simulink model "pd_plus_testings_7DOF_alternative"  (R2022b)
settings: Solver=ode4  StartTime=0.0  StopTime=101  FixedStep=1e-3  RelTol=1e-3
InitFcn:
  | parameters_7dof;
undefined symbols (not defined in the file): param_robot, q_0
(part 4 of 7)

== matlab function pd_plus_testings_7DOF_alternative/7 DOF Model/Mass Matrix1 ==
  data: q_state input; M output
function M = Franka_MassmMatrix(q_state)
% Author: TU Wien, ACIN Robotics group
% Optimized and generated from Maple

  M = zeros(7,7);
  t437 = q_state(6);
  t423 = sin(t437);
  t430 = cos(t437);
  t552 = 0.60149e-1 * t423 - 0.14117e-1 * t430;
  t302 = t552 + 0.384e0;
  t439 = q_state(4);
  t425 = sin(t439);
  t270 = t302 * t425;
  t440 = q_state(3);
  t433 = cos(t440);
  t327 = 0.60149e-1 * t430 + 0.14117e-1 * t423;
  t438 = q_state(5);
  t424 = sin(t438);
  t431 = cos(t438);
  t218 = t327 * t424 + 0.10517e-1 * t431;
  t426 = sin(t440);
  t484 = t218 * t426;
  t432 = cos(t439);
  t732 = 0.10517e-1 * t424;
  t495 = -t327 * t431 + t732;
  t965 = 0.825e-1 + t495;
  t974 = t432 * t965;
  t1004 = t484 + (t270 + t974) * t433;
  t436 = q_state(7);
  t422 = sin(t436);
  t355 = 0.12009367848960000000000000000000e-2 * t422;
  t275 = t355 + 0.63347540234880000000000000000000e-1;
  t429 = cos(t436);
  t379 = 0.29704261916160000000000000000000e-2 * t429;
  t190 = -t379 - t275;
  t361 = 0.55042935974400000000000000000000e-3 * t422;
  t408 = t422 ^ 2;
  t791 = 0.13297872941088000000000000000000e-4 * t408 + t361;
  t184 = 0.57804776249276620000000000000000e-2 + t791;
  t415 = t429 ^ 2;
  t375 = 0.24076459055801420000000000000000e-2 * t415;
  t516 = -t375 + t184;
  t615 = 0.79021743663150400000000000000000e-3 * t422;
  t865 = (-0.13614453378240000000000000000000e-2 + t615) * t429;
  t119 = t865 - t516;
  t992 = t119 * t423;
  t944 = t992 + t190;
  t1003 = t430 * t944;
  t232 = 0.10517000000000000000000000000000e-1 * t422 - 0.42520000000000000000000000000000e-2 * t429;
  t733 = 0.61597e-1 * t423;
  t556 = -0.10517e-1 * t429 - 0.4252e-2 * t422;
  t312 = -t556 + 0.88e-1;
  t854 = t312 * t430;
  t477 = t733 + t854;
  t955 = t424 * t477;
  t924 = -t232 * t431 + t955;
  t871 = t232 * t424;
  t818 = t430 * t431;
  t969 = -t312 * t818 - t431 * t733 + 0.825e-1;
  t126 = -t871 + t969;
  t476 = t312 * t423 - 0.61597e-1 * t430;
  t968 = 0.384e0 + t476;
  t948 = t425 * t968;
  t532 = -0.825e-1 + t948;
  t98 = t126 * t432 + t532;
  t1001 = t426 * t924 + t433 * t98;
  t975 = t965 * t425;
  t441 = q_state(2);
  t434 = cos(t441);
  t806 = t434 * t432;
  t427 = sin(t441);
  t822 = t427 * t433;
  t306 = t425 * t822 + t806;
  t857 = t306 * t430;
  t831 = t426 * t427;
  t807 = t434 * t425;
  t810 = t432 * t433;
  t298 = -0.1e1 * t427 * t810 + t807;
  t956 = t298 * t431;
  t201 = t424 * t831 + t956;
  t884 = t201 * t423;
  t979 = -0.1e1 * t884 + t857;
  t410 = t424 ^ 2;
  t417 = t431 ^ 2;
  t841 = t424 * t431;
  t672 = 0.4234e-2 * t841;
  t999 = 0.29474e-1 * t410 + 0.35549e-1 * t417 + t672 + 0.25853e-1;
  t998 = 0.28179e-1;
  t492 = 0.98827089590400000000000000000000e-3 * t422 + 0.52129746651620000000000000000000e-1;
  t198 = 0.24444132201840000000000000000000e-2 * t429 + t492;
  t997 = t198 * t423;
  t416 = t430 ^ 2;
  t523 = 0.33449653235675560000000000000000e-2 * t429 - 0.10967182128164640000000000000000e-2 * t422;
  t189 = 0.11022068765350630000000000000000e-1 + t523;
  t845 = t423 * t430;
  t779 = t189 * t845;
  t996 = (t119 * t416 - t779 + 0.23330419227411030000000000000000e-2) * t410;
  t364 = 0.25801376238000000000000000000000e-3 * t422;
  t290 = 0.13609823097337500000000000000000e-1 + t364;
  t384 = 0.63817750210500000000000000000000e-3 * t429;
  t939 = t384 + t290;
  t165 = t939 * t425;
  t995 = -t165 + t198;
  t590 = 0.10967182128164640000000000000000e-2 * t429;
  t324 = t423 * t590;
  t524 = -0.15804348732630080000000000000000e-2 * t415 - 0.13614453378240000000000000000000e-2 * t422 + 0.5826996021941340000000000000000e-3;
  t143 = (0.48418875570424600000000000000000e-2 * t422 + 0.55042935974400000000000000000000e-3) * t429 + t524;
  t959 = t143 * t430;
  t627 = -0.3030488946654060e-2 - t959;
  t994 = t324 + t627;
  t351 = 0.29704261916160000000000000000000e-2 * t422;
  t566 = 0.23898270415101870000000000000000e-1 - t351;
  t573 = 0.12009367848960000000000000000000e-2 * t429;
  t193 = t566 + t573;
  t376 = 0.79021743663150400000000000000000e-3 * t415;
  t292 = -0.68072266891200000000000000000000e-3 * t422 + 0.29134980109706700000000000000000e-3;
  t274 = 0.24209437785212300000000000000000e-2 * t422 + 0.27521467987200000000000000000000e-3;
  t866 = t274 * t429;
  t984 = t292 + t866;
  t967 = -t376 + t984;
  t987 = t967 * t423;
  t479 = -t987 - t193;
  t993 = t432 - 0.1e1;
  t610 = 0.33449653235675560000000000000000e-2 * t422;
  t105 = -(0.187138194629210e-3 + t610) * t423 - t994;
  t910 = t105 * t417;
  t991 = t218 * t433;
  t832 = t425 * t433;
  t741 = 0.4252e-2 * t429;
  t557 = 0.10517e-1 * t422 - t741;
  t513 = t557 * t431;
  t457 = t513 - t955;
  t990 = t457 * t426;
  t588 = 0.14820000000000000000000000000000e-2 * t429;
  t323 = t423 * t588;
  t612 = 0.23920000000000000000000000000000e-2 * t422;
  t849 = t422 * t429;
  t544 = 0.49780000000000000000000000000000e-2 * t849;
  t618 = 0.17120000000000000000000000000000e-2 * t415;
  t177 = t544 - 0.14600000000000000000000000000000e-2 - t618;
  t897 = t177 * t430;
  t799 = t897 - (0.682e-3 + t612) * t423;
  t930 = -t323 + 0.4234e-2 + t799;
  t989 = t841 * t930;
  t848 = t423 * t424;
  t988 = t848 * t967;
  t986 = t967 * t424;
  t985 = t967 * t430;
  t972 = t375 + t865;
  t115 = (-0.89033153705875550000000000000000e-2 - t791 + t972) * t416;
  t803 = t115 - t779;
  t402 = 0.345563e0 * t425;
  t389 = -0.825e-1 + t402;
  t551 = 0.41065e-1 * t424 + 0.11953e-1 * t431;
  t303 = t551 + 0.825e-1;
  t858 = t303 * t432;
  t203 = t389 + t858;
  t233 = -0.41065000000000000000000000000000e-1 * t431 + 0.11953000000000000000000000000000e-1 * t424;
  t129 = t203 * t426 + t233 * t433;
  t983 = -0.32797153116247448000000000000000e-1 - t791 + t865;
  t442 = q_state(1);
  t435 = cos(t442);
  t805 = t434 * t435;
  t763 = t426 * t805;
  t428 = sin(t442);
  t820 = t428 * t433;
  t982 = -t763 - t820;
  t592 = 0.54835910640823200000000000000000e-3 * t429;
  t325 = t423 * t592;
  t644 = t325 + 0.2390110552949070e-2;
  t613 = 0.16724826617837780000000000000000e-2 * t422;
  t856 = (0.93569097314605e-4 + t613) * t423;
  t981 = t910 + t644 + t856;
  t371 = 0.56786982094425000000000000000000e-2 * t425;
  t980 = -0.1e1 * t371 + 0.26431758938496000000000000000000e-1 * t432 + 0.21751134959804000000000000000000e-1;
  t769 = t431 * t831;
  t861 = t298 * t424;
  t183 = t861 - 0.1e1 * t769;
  t978 = -t996 - 0.1e1 * t361;
  t860 = t302 * t432;
  t976 = t425 * t495 - t860;
  t360 = 0.63817750210500000000000000000000e-3 * t422;
  t594 = 0.25801376238000000000000000000000e-3 * t429;
  t491 = 0.55993270925625000000000000000000e-2 + t594;
  t194 = -t360 + t491;
  t169 = t194 * t432;
  t483 = t592 + t613;
  t208 = t483 + 0.93569097314605e-4;
  t877 = t208 * t430;
  t281 = 0.56786982094425000000000000000000e-2 * t423 - 0.12089329343850000000000000000000e-2;
  t242 = t281 * t432;
  t164 = t423 * t939;
  t748 = 0.825e-1 * t434;
  t824 = t427 * t425;
  t973 = t748 * t810 + 0.825e-1 * t824;
  t546 = 0.85600000000000000000000000000000e-3 * t849;
  t617 = 0.24890000000000000000000000000000e-2 * t415;
  t221 = t546 + t617;
  t462 = t221 - 0.27050000000000000000000000000000e-2;
  t175 = t221 + 0.28220000000000000000000000000000e-2;
  t899 = t175 * t416;
  t460 = t899 + t462;
  t380 = 0.23920000000000000000000000000000e-2 * t429;
  t614 = 0.14820000000000000000000000000000e-2 * t422;
  t522 = -t380 + t614;
  t223 = -0.218e-3 + t522;
  t778 = t223 * t845;
  t101 = t778 + t460;
  t545 = 0.24890000000000000000000000000000e-2 * t849;
  t619 = 0.85600000000000000000000000000000e-3 * t415;
  t174 = t545 - 0.73000000000000000000000000000000e-3 - t619;
  t591 = 0.74100000000000000000000000000000e-3 * t429;
  t543 = t423 * t591;
  t744 = -0.11960000000000000000000000000000e-2 * t422 - 0.341e-3;
  t736 = t744 * t423 + 0.3449e-2;
  t971 = t101 * t841 + t174 * t430 - t543 + t736;
  t321 = 0.17120000000000000000000000000000e-2 * t849;
  t373 = 0.49780000000000000000000000000000e-2 * t415;
  t794 = t321 + t373;
  t800 = -t899 - t778;
  t509 = -0.33106000000000000000000000000000e-1 + t794 + t800;
  t804 = (-t462 + t800) * t417 - t989;
  t970 = t509 + t804;
  t124 = t375 + t983;
  t508 = -0.8292e-2 + t614;
  t179 = 0.5644000000000000000000000000000e-2 + t794;
  t784 = t179 * t845;
  t377 = 0.47840000000000000000000000000000e-2 * t429;
  t611 = 0.29640000000000000000000000000000e-2 * t422;
  t224 = t611 - t377 - 0.436e-3;
  t873 = t224 * t416;
  t966 = -0.1e1 * t508 + t380 + t873 - 0.1e1 * t784;
  t964 = -0.1e1 * t380 + t508 + t784 - 0.1e1 * t873;
  t458 = -t424 * t557 - t431 * t477;
  t569 = 0.11357396418885000000000000000000e-1 * t423 - 0.24178658687700000000000000000000e-2;
  t480 = t371 - 0.21751134959804000000000000000000e-1 * t432;
  t963 = t480 - 0.26431758938496000000000000000000e-1;
  t962 = -0.50330438027992300000000000000000e0 - t997;
  t961 = 0.29682175996164750000000000000000e0 + t164;
  t958 = t194 * t431;
  t607 = 0.88000000000000000000000000000000e-1 * t423;
  t279 = 0.38400000000000000000000000000000e0 + t607;
  t957 = t279 * t426;
  t548 = -0.104419e0 * t432 + 0.5317e-1 * t425;
  t953 = t427 * t548;
  t699 = 0.345563e0 * t432;
  t859 = t303 * t425;
  t626 = -t699 + t859;
  t952 = t427 * t626;
  t322 = t429 * t615;
  t816 = t430 * t433;
  t765 = t433 * t805;
  t830 = t426 * t428;
  t562 = t432 * (t765 - 0.1e1 * t830);
  t199 = 0.12763550042100000000000000000000e-2 * t429 + 0.51602752476000000000000000000000e-3 * t422 + 0.27219646194675000000000000000000e-1;
  t950 = (t199 * t430 + t569) * t431;
  t949 = (t626 - 0.316e0) * t434;
  t879 = t968 * t432;
  t277 = -t360 + 0.55993270925625000000000000000000e-2;
  t946 = (t277 + t594) * t432;
  t550 = -0.41065e-1 * t431 + 0.11953e-1 * t424;
  t945 = t550 * t426;
  t409 = t423 ^ 2;
  t365 = 0.31228377456598930000000000000000e-2 * t409;
  t789 = t365 - t322;
  t135 = 0.25022978729410880000000000000000e-2 * t415 + 0.81354094419858000000000000000000e-4 * t408 - t789 - 0.6284682367054690000000000000000e-3;
  t943 = t115 + t135;
  t229 = -0.825e-1 + t270;
  t941 = t229 + t974;
  t942 = t433 * t941 + t484;
  t382 = 0.13614453378240000000000000000000e-2 * t429;
  t790 = -t361 - t382;
  t388 = 0.54835910640823200000000000000000e-3 * t433;
  t595 = 0.24444132201840000000000000000000e-2 * t426;
  t938 = t388 + t595;
  t937 = -0.59408523832320000000000000000000e-2 * t422 + 0.24018735697920000000000000000000e-2 * t429 + 0.47796540830203740000000000000000e-1 + t143 * t423;
  t936 = -0.1e1 * t375 - 0.26431758938496000000000000000000e-1 * t430 - t983;
  t935 = t422 * t732 - t424 * t741 - t969;
  t353 = 0.15804348732630080000000000000000e-2 * t422;
  t287 = 0.24018735697920000000000000000000e-2 * t422 + 0.12669508046976000000000000000000e0;
  t464 = t287 + 0.59408523832320000000000000000000e-2 * t429;
  t885 = t199 * t423;
  t934 = ((0.66899306471351120000000000000000e-2 * t429 - 0.21934364256329280000000000000000e-2 * t422 + 0.22044137530701260000000000000000e-1) * t416 + ((0.48152918111602840000000000000000e-2 * t415 + (t353 - 0.27228906756480000000000000000000e-2) * t429 - 0.26595745882176000000000000000000e-4 * t408 - 0.11008587194880000000000000000000e-2 * t422 - 0.11560955249855324000000000000000e-1) * t423 - t464) * t430 - 0.52863517876992000000000000000000e-1 * t423 - 0.8968493211292842000000000000000e-2 - t523) * t431 + 0.27752814537092170000000000000000e0 + t885;
  t702 = 0.249498e0 * t427;
  t730 = 0.39252e-1 * t426;
  t933 = -t434 * t730 + t702;
  t673 = 0.7735484874e-2 * t429;
  t677 = 0.3127439544e-2 * t422;
  t932 = t673 + t677;
  t931 = 0.88e-1 * t430 + t733;
  t891 = t939 * t432;
  t927 = -t891 + t199;
  t354 = 0.12763550042100000000000000000000e-2 * t422;
  t291 = 0.11198654185125000000000000000000e-1 - t354;
  t593 = 0.51602752476000000000000000000000e-3 * t429;
  t926 = -0.1e1 * t593 - 0.1e1 * t291;
  t703 = 0.104419e0 * t425;
  t549 = 0.5317e-1 * t432 + t703;
  t304 = t549 - 0.825e-1;
  t502 = t304 * t426;
  t720 = 0.27454e-1 * t433;
  t925 = (t502 + t720) * t435;
  t923 = 0.735522e0 * t428;
  t701 = 0.735522e0 * t430;
  t381 = 0.16724826617837780000000000000000e-2 * t429;
  t362 = 0.54835910640823200000000000000000e-3 * t422;
  t567 = 0.44842466056464210000000000000000e-2 - t362;
  t191 = t381 + t567;
  t600 = 0.12089329343850000000000000000000e-2 * t425;
  t374 = 0.24209437785212300000000000000000e-2 * t415;
  t793 = t322 + t374;
  t898 = (0.31228377456598930000000000000000e-2 + t793) * t409;
  t922 = (t191 * t432 + t980 * t423 + t600 - 0.46305794820080000000000000000000e-2) * t431 + (0.23126197987767817000000000000000e-1 + t898) * t425;
  t706 = 0.27518e-1 * t428;
  t711 = 0.39252e-1 * t435;
  t921 = t435 * t702 + (-t434 * t711 - t706) * t426;
  t844 = t423 * t431;
  t920 = t174 * t844 + 0.8641e-2;
  t919 = -t177 * t844 - 0.17282e-1;
  t918 = 0.1225946e1 * t129;
  t352 = 0.24444132201840000000000000000000e-2 * t422;
  t489 = 0.98827089590400000000000000000000e-3 * t429 + 0.21447119530300000000000000000000e-1;
  t185 = -t352 + t489;
  t280 = -0.21751134959804000000000000000000e-1 * t423 + 0.46305794820080000000000000000000e-2;
  t916 = t185 * t424 + (-0.1e1 * t198 * t430 + t280) * t431;
  t915 = 0.25801376238000000000000000000000e-3 * t425 - 0.98827089590400000000000000000000e-3;
  t909 = t930 * t417;
  t914 = -t425 * t909 - 0.12805000000000000000000000000000e-1;
  t103 = (-0.1e1 * t865 + t516) * t423 - t190;
  t911 = t103 * t430;
  t571 = t306 * t423;
  t883 = t201 * t430;
  t136 = t571 + t883;
  t906 = t136 * t422;
  t905 = t136 * t429;
  t900 = (-0.99560000000000000000000000000000e-2 * t849 + 0.34240000000000000000000000000000e-2 * t415 + 0.29200000000000000000000000000000e-2) * t430;
  t160 = t179 * t416;
  t896 = t183 * t422;
  t895 = t183 * t429;
  t893 = t185 * t432;
  t892 = (-0.60427308755286430000000000000000e-2 + t790) * t409;
  t167 = t189 * t416;
  t192 = 0.89166132435286430000000000000000e-2 - t790;
  t890 = t192 * t432;
  t889 = t193 * t432;
  t888 = t194 * t425;
  t370 = 0.82500000000000000000000000000000e-1 * t425;
  t285 = 0.38400000000000000000000000000000e0 - t370;
  t197 = -t285 - 0.31600000000000000000000000000000e0 * t432;
  t887 = t197 * t430;
  t886 = t198 * t432;
  t202 = t483 + 0.9356909731460500000000000000000e-4;
  t882 = t202 * t424;
  t881 = t202 * t430;
  t880 = t203 * t433;
  t482 = -t590 - t610;
  t207 = -t482 + 0.187138194629210e-3;
  t878 = t207 * t423;
  t481 = -t588 - t612;
  t875 = (-t481 + 0.682e-3) * t430;
  t874 = t223 * t416;
  t225 = -t591 + t744;
  t872 = t225 * t430;
  t869 = t233 * t426;
  t272 = 0.18713819462921000000000000000000e-3 + t610;
  t868 = t272 * t423;
  t867 = t274 * t423;
  t864 = t277 * t425;
  t863 = t287 * t423;
  t246 = t292 * t423;
  t293 = 0.9356909731460500000000000000000e-4 + t613;
  t862 = t293 * t433;
  t853 = (0.47840000000000000000000000000000e-2 * t422 + 0.1364e-2) * t423;
  t847 = t423 * t426;
  t846 = t423 * t429;
  t843 = t424 * t426;
  t842 = t424 * t430;
  t840 = t424 * t432;
  t839 = t424 * t433;
  t838 = t424 * t434;
  t837 = t425 * t423;
  t836 = t425 * t424;
  t835 = t425 * t426;
  t834 = t425 * t430;
  t833 = t425 * t431;
  t828 = t426 * t432;
  t827 = t426 * t433;
  t826 = t426 * t434;
  t825 = t426 * t435;
  t823 = t427 * t432;
  t819 = t428 * t434;
  t817 = t430 * t432;
  t815 = t430 * t434;
  t814 = t431 * t432;
  t813 = t431 * t434;
  t812 = t432 * t423;
  t811 = t432 * t425;
  t809 = t433 * t434;
  t808 = t433 * t435;
  t715 = 0.10517e-1 * t435;
  t665 = t426 * t715;
  t721 = 0.10517e-1 * t433;
  t257 = -t428 * t721 - t434 * t665;
  t650 = t433 * t715;
  t728 = 0.10517e-1 * t428;
  t260 = -t426 * t728 + t434 * t650;
  t662 = t427 * t715;
  t802 = (-t260 * t425 + t432 * t662) * t423 + t257 * t842;
  t738 = 0.4252e-2 * t435;
  t267 = t738 * t809 - 0.4252e-2 * t830;
  t670 = t427 * t738;
  t740 = 0.4252e-2 * t430;
  t801 = (-t267 * t425 + t432 * t670) * t423 + t982 * t424 * t740;
  t181 = t224 * t845;
  t798 = t160 + t181;
  t757 = 0.88e-1 * t435;
  t685 = t433 * t757;
  t759 = 0.88e-1 * t426;
  t687 = t428 * t759;
  t268 = -t434 * t685 + t687;
  t686 = t427 * t757;
  t797 = t268 * t425 + t432 * t686;
  t368 = 0.35079000000000000000000000000000e-3 * t424;
  t283 = -t368 - 0.92549600000000000000000000000000e-3;
  t796 = t283 * t432 + t368;
  t574 = 0.10517000000000000000000000000000e-1 * t435;
  t795 = t574 * t826 + 0.10517000000000000000000000000000e-1 * t820;
  t746 = 0.825e-1 * t435;
  t401 = t433 * t746;
  t347 = t434 * t401;
  t406 = 0.316e0 * t427;
  t400 = t435 * t406;
  t792 = t347 + t400;
  t749 = 0.825e-1 * t433;
  t396 = t427 * t749;
  t788 = -t396 + 0.316e0 * t434;
  t787 = -0.1e1 * t432 + 0.1e1;
  t786 = -0.1e1 * t321 - 0.1e1 * t373;
  t785 = t432 * t898;
  t783 = t433 * t167;
  t154 = t189 * t812;
  t782 = t225 * t842;
  t333 = -0.8074e-2 * t431 - 0.458e-3 * t424;
  t781 = t333 * t811;
  t780 = t175 * t845;
  t153 = (0.21800000000000000000000000000000e-3 - t522) * t845;
  t776 = t424 * t813;
  t773 = t189 * t837;
  t772 = t430 * t807;
  t771 = t425 * t806;
  t770 = t426 * t819;
  t768 = t430 * t814;
  t767 = t431 * t810;
  t766 = t428 * t809;
  t764 = t435 * t824;
  t753 = 0.825e-1 * t428;
  t683 = t426 * t753;
  t762 = t432 * t683 + t792;
  t761 = -t406 + t973;
  t760 = -t425 * t748 + t788;
  t756 = 0.428e-3 * t422;
  t755 = 0.109e-3 * t423;
  t754 = 0.384e0 * t425;
  t752 = 0.384e0 * t428;
  t751 = 0.428e-3 * t429;
  t750 = 0.109e-3 * t430;
  t747 = 0.384e0 * t434;
  t745 = 0.384e0 * t435;
  t742 = 0.4252e-2 * t427;
  t739 = 0.3495e-2 * t435;
  t317 = -0.74100000000000000000000000000000e-3 * t422 + 0.4146e-2;
  t366 = 0.26431758938496000000000000000000e-1 * t423;
  t148 = -t366 - t191;
  t735 = t148 + t167;
  t336 = t425 * t662;
  t734 = t260 * t432 + t336;
  t731 = 0.27454e-1 * t426;
  t729 = 0.61597e-1 * t426;
  t727 = 0.14117e-1 * t428;
  t726 = 0.27454e-1 * t428;
  t725 = 0.39252e-1 * t428;
  t724 = 0.60149e-1 * t428;
  t719 = 0.27518e-1 * t433;
  t718 = 0.39252e-1 * t433;
  t717 = 0.61597e-1 * t433;
  t716 = 0.10517e-1 * t434;
  t714 = 0.14117e-1 * t435;
  t713 = 0.27454e-1 * t435;
  t712 = 0.27518e-1 * t435;
  t710 = 0.60149e-1 * t435;
  t709 = 0.61597e-1 * t435;
  t125 = t924 * t433;
  t624 = -0.1e1 * t854 - t733;
  t707 = 0.735522e0 * (t126 * t828 + t426 * t532 - t125) * t435 + (t1001 * t434 - 0.1e1 * t406 + (-t879 + (0.825e-1 - 0.1e1 * t871 + t624 * t431) * t425) * t427) * t923;
  t328 = 0.2872e-1 * t434 + 0.3141e-2 * t427;
  t704 = 0.646926e0 * t328;
  t128 = -t880 + t869;
  t697 = 0.1225946e1 * (t128 * t434 + t406 + (-0.1e1 * t859 + t699) * t427) * t435 + t428 * t918;
  t144 = -t945 + t880;
  t696 = 0.1225946e1 * (t144 * t434 - t406 + t952) * t428 + t435 * t918;
  t645 = t860 - t975;
  t695 = 0.1666555e1 * (t645 + 0.316e0) * t434 + 0.1666555e1 * t942 * t427;
  t137 = t426 * t712 + t428 * t933 + t433 * t711 + t706 * t809;
  t692 = 0.3228604e1 * t137;
  t630 = t304 * t433 - t731;
  t691 = -0.3587895e1 * t630 * t427 + 0.3587895e1 * (t548 - 0.316e0) * t434;
  t397 = t428 * t406;
  t680 = t426 * t746;
  t689 = t428 * t973 + t432 * t680 - t397;
  t681 = t433 * t747;
  t344 = t425 * t681;
  t688 = t344 + t761;
  t684 = t426 * t752;
  t682 = t428 * t748;
  t399 = t427 * t745;
  t679 = 0.3127439544e-2 * t279;
  t678 = 0.7735484874e-2 * t279;
  t676 = 0.3127439544e-2 * t424;
  t675 = 0.7735484874e-2 * t424;
  t674 = 0.3127439544e-2 * t429;
  t671 = t426 * t742;
  t669 = 0.15592e-1 * t811;
  t668 = 0.10517e-1 * t831;
  t667 = t428 * t729;
  t664 = t427 * t727;
  t663 = t427 * t724;
  t661 = t427 * t714;
  t660 = t427 * t710;
  t659 = t427 * t709;
  t658 = t428 * t716;
  t657 = t434 * t727;
  t656 = t434 * t724;
  t655 = t434 * t714;
  t654 = t434 * t712;
  t653 = t434 * t710;
  t652 = t434 * t709;
  t649 = 0.735522e0 * t832;
  t648 = t399 * t432 + t425 * t684 + t762;
  t642 = (0.76800000000000000000000000000000e0 * t423 + 0.17600000000000000000000000000000e0) * t673;
  t641 = t432 * t679;
  t286 = 0.31600000000000000000000000000000e0 - t370;
  t640 = t286 * t673;
  t639 = t344 * t428 + t745 * t835 + t689;
  t638 = t347 - t683;
  t637 = t765 - t830;
  t636 = t770 - t808;
  t635 = t735 + t1003;
  t632 = t770 - 0.1e1 * t808;
  t629 = -0.1e1 * t820 - 0.1e1 * t763;
  t628 = -0.1e1 * t766 - 0.1e1 * t825;
  t625 = t426 * t682 - t401;
  t623 = 0.7902174366315040000000000000000e-3 * t415;
  t622 = 0.2420943778521230000000000000000e-2 * t415;
  t621 = 0.5483591064082320000000000000000e-3 * t433;
  t616 = 0.28220000000000000000000000000000e-2 * t416;
  t609 = 0.14600000000000000000000000000000e-2 * t423;
  t608 = 0.49096519673609460000000000000000e-2 * t423;
  t606 = 0.86765250000000000000000000000000e-3 * t424;
  t605 = 0.42520000000000000000000000000000e-2 * t424;
  t604 = 0.49096519673609460000000000000000e-2 * t424;
  t602 = 0.54835910640823200000000000000000e-3 * t425;
  t601 = 0.63817750210500000000000000000000e-3 * t425;
  t598 = 0.25801376238000000000000000000000e-3 * t426;
  t597 = 0.63817750210500000000000000000000e-3 * t426;
  t596 = 0.16724826617837780000000000000000e-2 * t426;
  t589 = 0.11960000000000000000000000000000e-2 * t429;
  t586 = 0.54835910640823200000000000000000e-3 * t430;
  t585 = 0.16724826617837780000000000000000e-2 * t430;
  t584 = 0.11357396418885000000000000000000e-1 * t430;
  t583 = 0.54835910640823200000000000000000e-3 * t431;
  t582 = 0.25801376238000000000000000000000e-3 * t432;
  t581 = 0.54835910640823200000000000000000e-3 * t432;
  t580 = 0.63817750210500000000000000000000e-3 * t432;
  t579 = 0.16724826617837780000000000000000e-2 * t432;
  t578 = 0.49096519673609460000000000000000e-2 * t432;
  t577 = 0.10517000000000000000000000000000e-1 * t432;
  t572 = 0.21751134959804000000000000000000e-1 * t430;
  t570 = t322 - 0.60029938106866070000000000000000e-2;
  t568 = 0.12089329343850000000000000000000e-2 * t993;
  t563 = t432 * t632;
  t561 = -0.1e1 * t364 - 0.13609823097337500000000000000000e-1;
  t560 = t431 * t944 + t882;
  t559 = 0.2872e-1 * t427 - 0.3141e-2 * t434;
  t555 = t424 * t628;
  t554 = t425 * t629;
  t553 = t629 * t432;
  t547 = -t719 + t730;
  t542 = t423 * t598;
  t541 = t423 * t597;
  t540 = 0.49096519673609460000000000000000e-2 * t834;
  t539 = t423 * t581;
  t538 = t423 * t579;
  t537 = t431 * t578;
  t531 = t432 * t625 + t636 * t754 - t625;
  t162 = (-t427 * t746 - t435 * t681 + t684) * t425;
  t530 = (t399 - t638) * t432 + t162 + t400 + t638;
  t529 = 0.56786982094425000000000000000000e-2 * t787;
  t282 = -0.37417600000000000000000000000000e-3 + t606;
  t528 = t282 * t432 - t606;
  t519 = -0.1e1 * t384 + t561;
  t518 = t423 * t544;
  t507 = t366 + t381 + 0.44842466056464210000000000000000e-2 - t167 - 0.1e1 * t362;
  t506 = t376 - 0.1e1 * t866;
  t505 = -0.29640000000000000000000000000000e-2 * t846 + 0.8468e-2;
  t504 = -t589 + t780;
  t501 = (-t891 + t939) * t431 + t154;
  t500 = -0.65933151443131591200000000000000e0 - t642;
  t106 = t987 + (t293 + t592) * t430;
  t497 = t504 - t874;
  t494 = -t433 * t549 + t731;
  t490 = 0.11198654185125000000000000000000e-1 + t593;
  t487 = t425 * t551 - t699;
  t216 = t427 * t547 + 0.249498e0 * t434;
  t486 = t376 * t423 - 0.23898270415101870000000000000000e-1;
  t485 = t354 - t490;
  t236 = 0.16724826617837780000000000000000e-2 * t433 + 0.98827089590400000000000000000000e-3 * t426;
  t474 = t432 * t551 + t389;
  t473 = (0.12009367848960000000000000000000e-2 + t867) * t429 + t246 - t486;
  t470 = -(0.2489553776598930000000000000000e-3 + t793) * t416 + 0.23330419227411030000000000000000e-2 * t410 + 0.48418875570424600000000000000000e-2 * t415;
  t468 = 0.42520000000000000000000000000000e-2 * t982;
  t466 = -t432 * t678 + t601 - 0.24444132201840000000000000000000e-2;
  t463 = (0.104419e0 * t427 - 0.5317e-1 * t809) * t432 + (-0.104419e0 * t809 - 0.5317e-1 * t427) * t425;
  t461 = 0.46305794820080000000000000000000e-2 * t432 - t567 - t600;
  t459 = -t221 + 0.31784000000000000000000000000000e-1 + t798 + t804;
  t456 = t434 * t630 + t953;
  t455 = t425 * t552 + t432 * t495 - 0.825e-1;
  t454 = t945 + (-t402 - t858) * t433;
  t453 = t426 * t474 + t433 * t550;
  t452 = -t458 - 0.825e-1;
  t451 = t426 * t455 - t991;
  t450 = t487 * t427 + (t433 * t474 - t945) * t434;
  t449 = t425 * t458 - t879;
  t448 = t425 * t476 + t432 * t458 - 0.825e-1;
  t447 = (0.229e-3 + t872) * t431 + (-0.1e1 * t874 - 0.1e1 * t317 + t504) * t424 - t920;
  t446 = t976 * t427 + (t433 * t455 + t484) * t434;
  t445 = t426 * t448 + t433 * t457;
  t444 = t990 + (t432 * t452 - t948) * t433;
  t443 = t449 * t427 + (t433 * t448 - t990) * t434;
  t419 = t433 ^ 2;
  t418 = t432 ^ 2;
  t412 = t426 ^ 2;
  t411 = t425 ^ 2;
  t393 = t428 * t720;
  t385 = 0.21751134959804000000000000000000e-1 * t431;
  t372 = 0.54835910640823200000000000000000e-3 * t426;
  t348 = t425 * t686;
  t338 = t425 * t670;
  t337 = t433 * t654;
  t335 = t425 * t659;
  t332 = -0.8074e-2 * t424 + 0.458e-3 * t431;
  t319 = 0.458e-3 + t609;
  t310 = t434 * t713 - t753;
  t309 = t434 * t746 + t726;
  t308 = t434 * t726 + t746;
  t307 = t682 - t713;
  t300 = t574 * t824;
  t299 = t618 * t848;
  t288 = 0.82500000000000000000000000000000e-1 * t993;
  t284 = -0.31600000000000000000000000000000e0 * t425 + 0.82500000000000000000000000000000e-1;
  t269 = -t434 * t687 + t685;
  t265 = -t742 * t810 + 0.4252e-2 * t807;
  t264 = t433 * t709 - t434 * t667;
  t263 = -t433 * t658 - t665;
  t262 = -t426 * t652 - t428 * t717;
  t261 = t433 * t652 - t667;
  t259 = -t426 * t727 + t433 * t655;
  t258 = -t426 * t724 + t433 * t653;
  t256 = t426 * t655 + t433 * t727;
  t255 = t426 * t653 + t433 * t724;
  t254 = t426 * t714 + t433 * t657;
  t253 = -t426 * t710 - t433 * t656;
  t252 = t426 * t658 - t650;
  t251 = -t426 * t657 + t433 * t714;
  t250 = -t426 * t656 + t433 * t710;
  t249 = t425 * t716 - t721 * t823;
  t248 = t293 * t426;
  t245 = t290 * t425;
  t241 = t281 * t425;
  t234 = -t381 + t362;
  t231 = -0.12150e-1 * t841 - 0.4234e-2 * t410 + 0.4234e-2 * t417;
  t220 = t435 * t559 - 0.3495e-2 * t428;
  t213 = t285 * t673;
  t196 = -0.26431758938496000000000000000000e-1 * t425 - 0.56786982094425000000000000000000e-2 * t993;
  t188 = t286 + 0.38400000000000000000000000000000e0 * t432;
  t171 = t202 * t431;
  t170 = t464 * t423;
  t149 = -t197 + t607;
  t130 = t967 * t812;
  t127 = (-0.68072266891200000000000000000000e-3 * t429 - 0.27521467987200000000000000000000e-3 * t422 - 0.49096519673609460000000000000000e-2) * t430 + t234 * t423;
  t117 = (t261 * t425 + 0.88e-1 * t424 * t629 - t432 * t659) * t430;
  t108 = 0.42340000000000000000000000000000e-2 + t897 - t323 + (-0.68200000000000000000000000000000e-3 - t612) * t423;
  t107 = -t351 + t473;
  t91 = ((-0.68072266891200000000000000000000e-3 * t423 + t585 - 0.29704261916160000000000000000000e-2) * t429 + (-0.27521467987200000000000000000000e-3 * t423 - t586 - 0.12009367848960000000000000000000e-2) * t422 - t608) * t424 + (-0.25801376238000000000000000000000e-3 * t423 + (-0.12009367848960000000000000000000e-2 * t430 - 0.54835910640823200000000000000000e-3) * t431) * t429 + (0.63817750210500000000000000000000e-3 * t423 + (0.29704261916160000000000000000000e-2 * t430 - 0.16724826617837780000000000000000e-2) * t431) * t422;
  t90 = -t135 - t803;
  t86 = 0.15592e-1 + t964 * t431 - 0.1e1 * t299 + (t875 + t518 - 0.1e1 * t319) * t424;
  t82 = t936 * t431 + (t519 - t986) * t430 + (-t190 * t431 + t882 - 0.56786982094425000000000000000000e-2) * t423;
  t79 = (t507 - t1003) * t424 + (t881 - t479) * t431;
  t78 = ((t234 * t430 + t279 * t932 + t608) * t431 + (0.28244044800000000000000000000000e0 * t232 * t430 - 0.1e1 * t483) * t424) * t425 - 0.1e1 * t578 * t430 - 0.1e1 * t429 * t538 + t422 * t539 - 0.735522e0 * t556 * t288 * t431 + (t422 * t528 + t429 * t796) * t701;
  t77 = ((-0.1e1 * t190 * t423 + t936) * t424 + (-0.1e1 * t202 * t423 + t985) * t431) * t425 + ((t288 * t673 + t290 * t432 + t561) * t423 + t430 * t529) * t424 + t130 + t429 * t430 * t581 + t293 * t817;
  t70 = t416 * t890 + t501 * t430 + 0.23126197987767817000000000000000e-1 * t432 + t785 + (t423 * t529 + t425 * t635 + t568) * t431 + ((t106 + t193) * t425 + t946 - 0.1e1 * t594 - 0.1e1 * t277) * t424;
  t69 = (((-t430 * t579 - t466) * t431 + (-0.4252e-2 * t188 * t424 + 0.92549600000000000000000000000000e-3 * t425) * t701 - t424 * t581) * t429 + ((t641 + 0.5483591064082320000000000000000e-3 * t817 - t915) * t431 + (t188 * t732 + 0.37417600000000000000000000000000e-3 * t425) * t701 - t424 * t579) * t422 + t540) * t426 + (((-0.3127439544e-2 * t887 + 0.54835910640823200000000000000000e-3) * t431 - t424 * t585 + t149 * t675) * t429 + ((0.7735484874e-2 * t887 + 0.16724826617837780000000000000000e-2) * t431 + t424 * t586 + t149 * t676) * t422) * t433 + ((t381 * t425 - t422 * t602 + t537) * t426 + ((0.3127439544e-2 * t284 - t582) * t429 + (-0.7735484874e-2 * t284 + t580) * t422 + t604) * t433) * t423;
  t68 = ((-0.1e1 * t868 - 0.1e1 * t324 - t627) * t417 - t958 - t985 + t293 * t423 + t644) * t425 + ((t881 - 0.1e1 * t351 + t473) * t431 - 0.1644487577369270e-2) * t432 + (((-0.1e1 * t135 - t803) * t431 - t939 * t430 - 0.1e1 * t281) * t425 + (-0.1e1 * t167 + t911 - 0.1e1 * t148) * t432) * t424;
  t67 = (((-0.1e1 * t198 * t431 - 0.56786982094425000000000000000000e-2) * t432 + (-t285 * t677 - t213 - 0.63347540234880000000000000000000e-1) * t431 - 0.1e1 * t882 + 0.56786982094425000000000000000000e-2) * t423 + ((t385 + t519) * t432 + (-0.1e1 * t371 + 0.26431758938496000000000000000000e-1) * t431 + t986 + 0.13609823097337500000000000000000e-1 + t932 * t284) * t430 + t124 * t431) * t433 + (((-0.1e1 * t190 * t424 - t171) * t432 + (t286 * t677 + t640 + 0.52129746651620000000000000000000e-1) * t424) * t423 + ((t431 * t967 - 0.26431758938496000000000000000000e-1 * t424) * t432 + (t371 - 0.21751134959804000000000000000000e-1) * t424) * t430 - t124 * t840) * t426 + (((0.13609823097337500000000000000000e-1 * t431 - 0.21751134959804000000000000000000e-1) * t423 - 0.52129746651620000000000000000000e-1 * t430) * t433 + ((-t292 - 0.13609823097337500000000000000000e-1 * t424 + t506) * t423 - t881) * t426) * t425;
  t64 = ((((t236 * t432 - 0.1e1 * t425 * t598 + 0.12009367848960000000000000000000e-2 * t426) * t430 + t372 + t466 * t433) * t431 + (t283 * t649 + (-0.1e1 * t596 + (0.12009367848960000000000000000000e-2 * t432 + 0.98827089590400000000000000000000e-3) * t433) * t424) * t430 + (t424 * t938 - 0.1e1 * t542) * t432 + (-0.1e1 * t236 * t423 - 0.1e1 * t424 * t597) * t425 + t675 * t957 + t542) * t429 + (((-0.1e1 * t432 * t621 + (-0.24444132201840000000000000000000e-2 * t432 + t601 - 0.29704261916160000000000000000000e-2) * t426) * t430 + t596 + (-0.1e1 * t641 + t915) * t433) * t431 + (t282 * t649 + (t372 + (-0.29704261916160000000000000000000e-2 * t432 - 0.24444132201840000000000000000000e-2) * t433) * t424) * t430 + (t236 * t424 + t541) * t432 + (t423 * t938 - 0.1e1 * t424 * t598) * t425 + t676 * t957 - 0.1e1 * t541) * t422 - 0.1e1 * t423 * t433 * t537 - 0.1e1 * t433 * t540 + t604 * t847) * t427 + (0.49096519673609460000000000000000e-2 * t423 * t833 - 0.49096519673609460000000000000000e-2 * t817 + ((t425 * t678 + t580 - 0.63817750210500000000000000000000e-3) * t431 + (-0.16327680000000000000000000000000e-2 * t836 + t796) * t701 - 0.1e1 * t424 * t602 - 0.1e1 * t585 * t833 - 0.1e1 * t538) * t429 + ((t425 * t679 + t582 - 0.25801376238000000000000000000000e-3) * t431 + (0.40385280000000000000000000000000e-2 * t836 + t528) * t701 - 0.16724826617837780000000000000000e-2 * t836 + t583 * t834 + t539) * t422) * t434;
  t63 = ((t189 * t814 + (-t382 - 0.1e1 * t361 - 0.89166132435286430000000000000000e-2) * t425) * t416 + ((t245 - t492 - t640) * t431 - 0.1e1 * t773 + t560 * t432) * t430 + (t286 * t674 + t130 - t352 - t864 + t889 + 0.21447119530300000000000000000000e-1) * t424 - t922) * t426 + t424 * t783 + (-t171 + (t992 - t213 + t245 - t275 - t886) * t424) * t816 + ((-t285 * t674 - t566 + t864 - t893 - t987) * t431 + (t423 * t963 - t381 + t461) * t424) * t433;
  t62 = (((-0.1e1 * t372 * t429 - 0.1e1 * t248 + (t190 * t432 - t995) * t433) * t424 + (-0.56786982094425000000000000000000e-2 * t426 + ((-0.1e1 * t595 + t621) * t429 - t492 * t426 + t862) * t431) * t432 + ((t431 * t939 - 0.21751134959804000000000000000000e-1) * t426 + t967 * t433) * t425 + (-0.1e1 * t275 * t431 + 0.56786982094425000000000000000000e-2) * t426) * t423 + (t426 * t985 + (t124 * t432 + t430 * t980) * t433) * t424 + ((t388 * t429 + t862) * t425 + (t623 - 0.1e1 * t866 - 0.1e1 * t292) * t767 + ((t385 + t561) * t432 + (-0.56786982094425000000000000000000e-2 * t431 - 0.1e1 * t198) * t425 + 0.26431758938496000000000000000000e-1 * t431 + t787 * t384 + t290) * t426) * t430) * t427 + t434 * ((-0.1e1 * t190 * t425 + t891 - 0.1e1 * t939) * t424 + t967 * t432 + (-0.5483591064082320000000000000000e-3 * t429 - 0.1e1 * t293) * t833) * t423 + (-t124 * t425 + t196 * t430) * t838 + (t202 * t432 + (-0.1e1 * t623 + t984) * t833) * t815 + (-0.1e1 * t379 * t423 + t124) * t769;
  t61 = (-t430 * t891 - t242) * t843 + ((t105 * t431 + t169 + t485) * t424 + (t374 + t570) * t417 + (t430 * t927 - t242 + t569) * t431 + (-0.1e1 * t371 + 0.52863517876992000000000000000000e-1) * t430 - 0.1e1 * t863 + t500 + t978) * t433 + ((t90 * t841 - 0.1e1 * t958 - t985 + t981) * t426 + (t572 + t962) * t433) * t432 + ((((-t379 - 0.1e1 * t355 - 0.63347540234880000000000000000000e-1 + (-0.1e1 * t184 + t972) * t423) * t430 + t735) * t424 + (-0.1e1 * t877 + (-0.1e1 * t867 - 0.12009367848960000000000000000000e-2) * t429 - 0.1e1 * t246 + t351 + t486) * t431 + 0.1644487577369270e-2) * t426 + (t916 + t961) * t433) * t425;
  t60 = ((t192 * t832 + (-0.1e1 * t767 + t843) * t189) * t416 - 0.1e1 * t248 * t818 - t810 * t988 + ((-0.1e1 * t429 * t583 + (t992 + t165 - 0.1e1 * t886 - 0.1e1 * t379 - 0.1e1 * t275) * t424) * t430 + ((-0.1e1 * t292 + t506) * t423 - 0.1e1 * t893 + t888 - 0.1e1 * t573 - 0.1e1 * t566) * t431 + t963 * t848 + (t461 - 0.1e1 * t381) * t424) * t426 + ((t995 * t431 + t773 + ((-t992 - 0.1e1 * t190) * t431 - 0.1e1 * t882) * t432) * t430 + (-0.1e1 * t889 + t888 - 0.1e1 * t185) * t424 + t922) * t433) * t427 + (t425 * t560 + t501) * t815 + (-0.1e1 * t191 * t425 + t196 * t423 + t568) * t813 + t807 * t988 + (t193 * t425 + t169 - 0.1e1 * t194) * t838 + 0.23126197987767817000000000000000e-1 * t806 + ((t189 * t833 + t890) * t416 + t785) * t434;
  t59 = (-0.36044563611157510600000000000000e0 + ((t207 * t424 - 0.11357396418885000000000000000000e-1) * t430 + t937 * t424 + t934) * t418 + (0.56786982094425000000000000000000e-2 * t430 - t164 + 0.12908973617152500000000000000000e-1 + t916) * t432 + ((-t165 - t944) * t430 - 0.1e1 * t241 + t507) * t431 + (-0.1e1 * t208 * t424 + 0.56786982094425000000000000000000e-2) * t430 + t479 * t424 - t164 + (((-0.1e1 * t365 - 0.28801560650267140000000000000000e-2 + t793 + t803) * t417 + ((t143 * t424 + t199) * t430 + (-0.1e1 * t878 + 0.3030488946654060e-2) * t424 + t569) * t431 + (-0.1e1 * t189 * t423 - 0.52863517876992000000000000000000e-1) * t430 + t485 * t424 - 0.1e1 * t892 + t170 - 0.1e1 * t429 * t353 + 0.54368101124215626900000000000000e0 - 0.1e1 * t470) * t432 - 0.1e1 * t572 + t194 * t424 + t997 + 0.58416762559717300000000000000000e0) * t425) * t426 + ((-0.1e1 * t877 + t479) * t431 + 0.1644487577369270e-2 + t635 * t424) * t810 + ((t424 * t939 + t967) * t425 - 0.1e1 * t198 * t424) * t816 + t280 * t839 + ((t627 + t878) * t417 - 0.1e1 * t208 * t423 + t281 * t424 - 0.2390110552949070e-2) * t832 + (((-0.1e1 * t360 + (-0.1e1 * t779 + t943) * t424 + t491) * t425 - 0.1e1 * t185) * t431 - 0.13297019103287584000000000000000e-1) * t433;
  t58 = (((-0.1e1 * t154 * t816 + (-0.3344965323567556e-2 * t422 - 0.187138194629210e-3) * t847) * t424 + t832 * t877 + (t107 * t425 + t169) * t433) * t431 + (t891 * t816 + (-0.1e1 * t783 + t103 * t816 - 0.1e1 * t148 * t433) * t425) * t424 - 0.16444875773692700000000000000000e-2 * t832 - 0.1e1 * t287 * t847 + (-0.1e1 * t910 + t985 - 0.1e1 * t856 - 0.1e1 * t325 - 0.23901105529490700000000000000000e-2 + (t431 * t943 + t281) * t424) * t810) * t427 + ((t107 + t877) * t432 + (t424 * t90 - 0.1e1 * t194) * t425) * t813 + (-0.1e1 * t165 * t430 - 0.1e1 * t241 + (-0.1e1 * t735 + t911) * t432) * t838 - 0.1e1 * t967 * t772 - 0.1644487577369270e-2 * t806 + t981 * t807 + ((t622 + 0.790217436631504e-3 * t849 - 0.6002993810686607000000000000000e-2) * t417 + ((((0.4841887557042460e-2 * t422 + 0.55042935974400000000000000000000e-3) * t429 + t524) * t430 - 0.1096718212816464e-2 * t846 + 0.3030488946654060e-2) * t424 + (-t198 * t425 + t927) * t430 - 0.1e1 * t242 + t280 * t425 + t569) * t431 + (t926 + t946 + (-0.1e1 * t352 + t489) * t425) * t424 + (-0.1e1 * t480 + 0.52863517876992000000000000000000e-1) * t430 + t962 * t432 + t961 * t425 - 0.1e1 * t642 - 0.65933151443131591200000000000000e0 + t978) * t831;
  t57 = ((t706 + 0.39252000000000000000000000000000e-1 * t805) * t433 + (0.27518000000000000000000000000000e-1 * t805 - 0.1e1 * t725) * t426) * t692 + 0.3228604e1 * ((-0.39252000000000000000000000000000e-1 * t426 + t719) * t435 + (-0.27518000000000000000000000000000e-1 * t426 - 0.1e1 * t718) * t819) * ((-0.27518e-1 * t426 - 0.1e1 * t718) * t428 + t337 + t933 * t435) + (t129 * t805 + (-0.1e1 * t869 + t880) * t428) * t696 + (t128 * t435 + t129 * t819) * t697 + ((t426 * t98 - 0.1e1 * t125) * t805 + t1001 * t428) * t707 + 0.735522e0 * (((t430 * t734 + t468) * t431 + (-0.1e1 * t764 + (-0.1e1 * t765 + t830) * t432) * t605 + t802) * t429 + (((t267 * t432 + t338) * t430 + t795) * t431 + (t300 + 0.10517000000000000000000000000000e-1 * t562) * t424 + t801) * t422 + ((t261 * t432 + t335) * t431 + t262 * t424 + t797) * t423 + (-0.1e1 * t268 * t432 + t348) * t818 + t117 + t530) * ((t263 * t842 + (-0.1e1 * t768 + t837) * t252 + 0.42520000000000000000000000000000e-2 * t628 * t431 + t563 * t605) * t429 + (-0.4252e-2 * (-0.1e1 * t837 + t768) * t636 + t555 * t740 + 0.10517000000000000000000000000000e-1 * (t766 + t825) * t431 + (-0.1e1 * t770 + t808) * t424 * t577) * t422 + (t264 * t814 - 0.1e1 * t269 * t425 + 0.61597e-1 * t555) * t423 + t269 * t768 + (t264 * t425 + 0.88e-1 * t555) * t430 + t531) + (t970 * t832 * t432 + t971 * t835 + (-0.1e1 * t619 + t545) * t423 * t839 + (t432 * t447 + t914) * t426 + ((t966 * t431 + t299 - 0.15592e-1 + (-0.1e1 * t875 - 0.1e1 * t518 + t319) * t424) * t418 + (-0.1e1 * t317 + t497) * t431 - 0.1e1 * t782 + 0.19192000000000000000000000000000e-1 + (-0.73000000000000000000000000000000e-3 * t423 - 0.229e-3) * t424) * t433) * t427 + t86 * t771 + t108 * t411 * t776 + ((-0.1e1 * t546 - 0.1e1 * t617) * t410 + (-0.1e1 * t221 * t417 + t509) * t418 + (-0.27050000000000000000000000000000e-2 + t899 - 0.1e1 * t153) * t411 * t417 + 0.84106000000000000000000000000000e-1) * t434 + 0.3587895e1 * (-0.1e1 * t310 * t433 + t309 * t426 + 0.104419e0 * t554 + 0.5317e-1 * t553) * (t307 * t433 + t397 + (-0.1e1 * t549 * t435 + t308) * t426 + t463 * t428) + 0.3587895e1 * (t309 * t433 + t400 + (t428 * t549 + t310) * t426 + t463 * t435) * (t308 * t433 - 0.1e1 * t307 * t426 + t632 * t703 + 0.5317e-1 * t563) + 0.1666555e1 * ((t250 * t424 + (t425 * t663 - 0.1e1 * t253 * t432) * t431 + t254 * t425 - 0.1e1 * t432 * t664) * t430 + (t251 * t424 + (t254 * t432 + t425 * t664) * t431 + t253 * t425 + t432 * t663) * t423 + (t263 * t432 - 0.1e1 * t728 * t824) * t424 - 0.1e1 * t252 * t431 + t397 + t628 * t754 + t752 * t823 + t787 * t680 + (-0.1e1 * t824 + t787 * t809) * t753) * ((t255 * t814 + t256 * t425 + t258 * t424) * t430 + (t256 * t814 - 0.1e1 * t255 * t425 + t259 * t424) * t423 + t257 * t840 + t260 * t431 + 0.384e0 * t554 + 0.825e-1 * t553 + t434 * t680 + t428 * t749) + 0.1666555e1 * ((-0.1e1 * t255 * t424 + (t258 * t432 + t425 * t660) * t431 + t259 * t425 - 0.1e1 * t432 * t661) * t430 + (-0.1e1 * t256 * t424 + (t259 * t432 + t425 * t661) * t431 - 0.1e1 * t258 * t425 + t432 * t660) * t423 - 0.1e1 * t734 * t424 + t257 * t431 + t530) * ((t250 * t814 + t251 * t425 + t253 * t424) * t430 + (-0.1e1 * t250 * t425 + t251 * t814 - 0.1e1 * t254 * t424) * t423 + t252 * t840 + t263 * t431 + t531);
  t56 = (((t249 * t430 + t671) * t431 - 0.1e1 * t265 * t424 + t668 * t842 + 0.10517e-1 * t571) * t429 + ((t265 * t430 - 0.1e1 * t668) * t431 + t249 * t424 + t671 * t842 + 0.4252e-2 * t571) * t422 + (t424 * t427 * t759 - 0.1e1 * t717 * t824 - 0.61597e-1 * t806) * t430 + t427 * t729 * t848 + 0.88e-1 * t571 + (0.384e0 * t822 - 0.1e1 * t748) * t425 + (t396 + t747) * t432 + t788 + t931 * t956) * ((((t336 + 0.10517e-1 * t562) * t430 + t468) * t431 + (-0.1e1 * t637 * t432 - 0.1e1 * t764) * t605 + t802) * t429 + ((t338 * t430 + t562 * t740 + t795) * t431 + (t577 * t637 + t300) * t424 + t801) * t422 + (t335 * t423 + t348 * t430 + t562 * t931) * t431 + t117 + t262 * t848 + t797 * t423 + t162 + (t432 - 0.1e1) * t683 + (t399 - 0.1e1 * t347) * t432 + t792) * t923 + (0.95220000000000000000000000000000e-2 + (-0.6898e-2 + (-0.1e1 * t900 - 0.1e1 * t853 + t505) * t417 + (-0.1e1 * t181 - 0.1e1 * t160 + 0.5410000000000000000000000000000e-2 + t786) * t841 + t323 - 0.1e1 * t799) * t432 + ((-0.1e1 * t875 + 0.458e-3) * t431 + t964 * t424 + t919) * t425) * t427 * t419 + ((t418 * t970 + t811 * t86 + t459) * t831 + t447 * t806 + t425 * t101 * t776 + t174 * t772 - 0.1e1 * t543 * t807 + (t425 * t736 + t914) * t434) * t433 + (-0.15015000000000000000000000000000e-1 + (-t909 + t971) * t432 + ((-0.1e1 * t872 - 0.229e-3) * t431 + (t874 - 0.1e1 * t780 + t589 + t317) * t424 + t920) * t425) * t427 - 0.704e-3 * t434 + ((t101 * t417 + t989 - 0.1e1 * t509) * t771 + (-0.1e1 * t497 + t317) * t813) * t426 + (t86 * t418 + t782 - 0.19192000000000000000000000000000e-1 + (-0.1e1 * t174 * t423 + 0.229e-3) * t424) * t826 + (t220 * t704 + 0.3228604e1 * ((t654 - 0.1e1 * t725) * t433 + t921) * t216 - 0.1e1 * (t304 * t830 + t393) * t691 - 0.1e1 * ((-0.1e1 * t880 + t945) * t427 + t949) * t697 + (-0.1e1 * t218 * t820 + 0.1e1 * t965 * t428 * t828 + t229 * t830) * t695) * t428 + (-0.1e1 * t739 * t704 - 0.1e1 * t216 * t692 - 0.1e1 * t925 * t691 + (t144 * t427 - 0.1e1 * t949) * t696 - 0.1e1 * ((t432 * t935 - t532) * t822 + (-0.1e1 * t425 * t935 - t879 - 0.316e0) * t434 + (t424 * t624 + t513) * t831) * t707 + (-0.1e1 * t991 + t426 * t941) * t695 * t435 + (-0.1e1 * t559 * t704 + ((t942 + (-t974 - 0.1e1 * t270 + 0.825e-1) * t433 - 0.1e1 * t484) * t434 + (0.1e1 * t975 - 0.1e1 * t860 + t645) * t427) * t695) * t428) * t435;
  M(7,3) = t78;
  M(4,1) = t58;
  M(6,3) = t77;
  M(1,1) = (0.4815e-2 * t884 - 0.4815e-2 * t857 - 0.1196e-2 * t905 - 0.1196e-2 * t896 + 0.741e-3 * t906 - 0.741e-3 * t895) * (t884 - 0.1e1 * t857) + (0.1964e-2 * t883 + 0.1964e-2 * t571 - 0.1e1 * t201 * t755 + t306 * t750 + 0.1158e-2 * t769 - 0.1158e-2 * t861) * t136 + (-0.5433e-2 * t769 + 0.5433e-2 * t861 - 0.1158e-2 * t883 - 0.1158e-2 * t571 + 0.341e-3 * t979) * t183 + (0.12516e-1 * t905 + 0.12516e-1 * t896 + t136 * t756 - 0.1e1 * t183 * t751 + 0.1196e-2 * t979) * (t896 + t905) + (-0.10027e-1 * t906 + 0.10027e-1 * t895 - 0.1e1 * t136 * t751 - 0.1e1 * t183 * t756 + 0.741e-3 * t979) * (-0.1e1 * t906 + t895) + 0.17079e-1 + (-0.4354e-2 * t884 + 0.4354e-2 * t857 + t201 * t750 + t306 * t755 + 0.341e-3 * t183) * t979 + 0.4970684e1 * (-0.3875e-2 * t428 - 0.2081e-2 * t435) ^ 2 + 0.4970684e1 * (0.3875e-2 * t435 - 0.2081e-2 * t428) ^ 2 + 0.3587895e1 * (t428 * t456 - t397 + t925) ^ 2 + 0.3587895e1 * (t393 + t428 * t502 + (t434 * t494 - t953) * t435 + t792) ^ 2 + 0.3228604e1 * t137 ^ 2 + 0.3228604e1 * (-t428 * t718 + t337 + t921) ^ 2 + 0.1666555e1 * (t428 * t446 + t435 * t451 + t639) ^ 2 + 0.1666555e1 * (t451 * t428 + ((t432 * t552 - t975) * t427 - t1004 * t434) * t435 + t648) ^ 2 + 0.1225946e1 * (t428 * t450 + t435 * t453 + t689) ^ 2 + 0.1225946e1 * (t453 * t428 + (t434 * t454 - t952) * t435 + t762) ^ 2 + 0.735522e0 * (t428 * t443 + t435 * t445 + t639) ^ 2 + 0.735522e0 * (t445 * t428 + ((t425 * t452 + t432 * t476) * t427 + t444 * t434) * t435 + t648) ^ 2 + 0.646926e0 * (-t428 * t559 - t739) ^ 2 + 0.646926e0 * t220 ^ 2 + (0.30978000000000000000000000000000e-1 + t669 + t781 + t998 * t418 + t999 * t411) * t434 ^ 2 + ((-0.1e1 * (-0.2664e-2 * t425 + 0.17282e-1 * t432) * t426 - 0.7850e-2 + t332 * t828 - 0.1e1 * t231 * t835 - 0.25610000000000000000000000000000e-1 * t426 + (0.15592e-1 * t411 - 0.15592e-1 * t418 + (-0.1e1 * t418 + t411) * t333 + 0.22792000000000000000000000000000e-1 + (0.4652e-2 - 0.58948e-1 * t410 - 0.71098e-1 * t417 - 0.8468e-2 * t841) * t811) * t433) * t434 + (0.36155000000000000000000000000000e-1 + (0.28323e-1 + 0.35549e-1 * t410 + 0.29474e-1 * t417 - 0.1e1 * t672) * t412 + (0.95220000000000000000000000000000e-2 + (-0.2664e-2 + t231) * t432 + (-0.17282e-1 + t332) * t425) * t827 + (-0.1e1 * t669 + 0.1087000000000000000000000000000e-2 - 0.1e1 * t781 + t999 * t418 + t998 * t411) * t419) * t427) * t427;
  M(5,4) = t79;
  M(7,5) = t127;
  M(3,7) = t78;
  M(5,6) = t106;
  M(5,1) = t60;
  M(2,5) = t63;
  M(2,3) = t59;
  M(4,4) = t996 + (-0.1e1 * t354 + (t868 + t994) * t431 + t490) * t424 + (-t199 * t431 - 0.52863517876992000000000000000000e-1) * t430 + (-t570 - t622) * t417 - t569 * t431 + t863 + t361 - t500;
  M(1,5) = t60;
  M(4,6) = t82;
  M(6,5) = t106;
  M(7,4) = t91;
  M(5,7) = t127;
  M(7,7) = 0.49096519673609460000000000000000e-2;
  M(6,7) = -t483;
  M(1,6) = t62;
  M(3,4) = t68;
  M(2,2) = 0.3228604e1 * (t434 * t547 - t702) ^ 2 + 0.3587895e1 * (-t406 + t456) ^ 2 + 0.646926e0 * t559 ^ 2 + 0.1666555e1 * (t446 + t688) ^ 2 + 0.735522e0 * (t443 + t688) ^ 2 + ((-0.1e1 * t778 - 0.1e1 * t616) * t418 + t459) * t419 + ((0.33106000000000000000000000000000e-1 + (-0.1e1 * t153 + t460) * t417 + t221 * t416 + t786) * t418 + (-0.15592000000000000000000000000000e-1 + ((-0.1e1 * t377 - 0.43600000000000000000000000000000e-3 + t611) * t416 + (-0.56440000000000000000000000000000e-2 + t786) * t845 + 0.82920000000000000000000000000000e-2 - 0.1e1 * t522) * t431 + t299) * t811 + (t108 * t431 * t418 + ((t481 - 0.68200000000000000000000000000000e-3) * t430 + t609 + 0.45800000000000000000000000000000e-3 - 0.1e1 * t518) * t811) * t424) * t412 + 0.10340700000000000000000000000000e0 + (-0.9522e-2 + (0.6898e-2 + (-0.1e1 * t505 + t853 + t900) * t417 + (-0.5410000000000000000000000000000e-2 + t794 + t798) * t841 - 0.1e1 * t323 + t799) * t432 + ((-0.458e-3 + t875) * t431 + t966 * t424 - 0.1e1 * t919) * t425) * t827 + 0.1225946e1 * (t450 + t761) ^ 2 + (t153 - 0.1e1 * t616) * t411 + t221 * t409 + (t428 ^ 2 + t435 ^ 2) * (0.3587895e1 * (t427 * t494 + t434 * t548 - t788) ^ 2 + 0.3228604e1 * t216 ^ 2 + 0.735522e0 * (t427 * t444 + t434 * t449 - t760) ^ 2 + 0.1666555e1 * (t1004 * t427 - t434 * t976 + t760) ^ 2 + 0.1225946e1 * (-t427 * t454 - t434 * t487 + t760) ^ 2 + 0.646926e0 * t328 ^ 2);
  M(2,7) = t69;
  M(7,2) = t69;
  M(1,3) = t57;
  M(5,2) = t63;
  M(3,2) = t59;
  M(5,5) = (0.3122837745659893e-2 + t793) * t409 + t779 + t192 * t416 + 0.23126197987767817000000000000000e-1;
  M(3,1) = t57;
  M(3,5) = t70;
  M(2,6) = t67;
  M(4,3) = t68;
  M(2,1) = t56;
  M(7,6) = -t483;
  M(4,7) = t91;
  M(1,4) = t58;
  M(4,5) = t79;
  M(1,2) = t56;
  M(6,6) = -t374 - t865 + t361 + 0.32810450989188536000000000000000e-1;
  M(2,4) = t61;
  M(6,1) = t62;
  M(5,3) = t70;
  M(1,7) = t64;
  M(6,2) = t67;
  M(4,2) = t61;
  M(6,4) = t82;
  M(7,1) = t64;
  M(3,6) = t77;
  M(3,3) = 0.69005519272293457500000000000000e0 + ((-0.1e1 * t374 + 0.175156065026714e-3 + t789) * t417 - 0.1e1 * t950 + t779 + t892 + (t353 + 0.51602752476000000000000000000000e-3 * t424) * t429 + t291 * t424 - 0.53893925569918450000000000000000e0 + t470) * t418 + ((-0.1e1 * t584 + t934) * t425 + t950 - 0.80863245317250000000000000000000e-1 + (((t272 + t590) * t430 + t937) * t425 + t926) * t424) * t432 + ((-0.27050000000000000000000000000000e-2 + t803) * t417 + (t959 + (t482 - 0.18713819462921000000000000000000e-3) * t423 + 0.30304889466540600000000000000000e-2) * t841 - 0.52863517876992000000000000000000e-1 * t430 + t170 + 0.4741755542971769000000000000000e-2) * t411 + (t584 - 0.1e1 * t885 - 0.28391278634449500000000000000000e0) * t425 + (0.3122837745659893e-2 * t416 + 0.2333041922741103e-2) * t417 + (-0.1e1 * t374 - 0.1e1 * t322 + 0.32979938106866070000000000000000e-2) * t410 - t790;
end

== matlab function pd_plus_testings_7DOF_alternative/7 DOF Model/MATLAB Function ==
  data: q input; q_pp output; q_p input; tau input; M input; C input; g input
function q_pp = fcn(q,q_p,tau,M,C,g)

q_pp = M\(tau - C*q_p - g);

== matlab function pd_plus_testings_7DOF_alternative/Subsystem/Robot model bus ==
  settings: updateMethod=DISCRETE  sampleTime=param_global.Ta
  data: q input; q_p input; q_pp input; H input; J input; J_p input; M input; C_rnea input; C input; g input; robot_model output Bus: robot_model
function robot_model = fcn(q, q_p, q_pp, H, J, J_p, M, C_rnea, C, g)
% Parameters
robot_model=struct();
robot_model.q=q;                    % generalized coordinates
robot_model.q_p=q_p;                % time derivative of generalized coordinates
robot_model.q_pp=q_pp;
robot_model.H=H;
robot_model.J=J;
robot_model.J_p=J_p;
robot_model.M=M;
robot_model.C_rnea=C_rnea; % C_rnea(q, q_p) = C(q, q_p)q_p + g(q) = n(q, q_p)
robot_model.C=C;
robot_model.g=g;
end
